simulink model "UnoANFIS"  (R2017a)
settings: Solver=VariableStepAuto  StartTime=0.0  StopTime=1299  RelTol=1e-3
undefined symbols (not defined in the file or in its folder): anfis, anfis3, datos2
libraries: dspsrcs4 x4, fuzblock x1
settings Model: Creator=Dell  LastModifiedBy=Dell

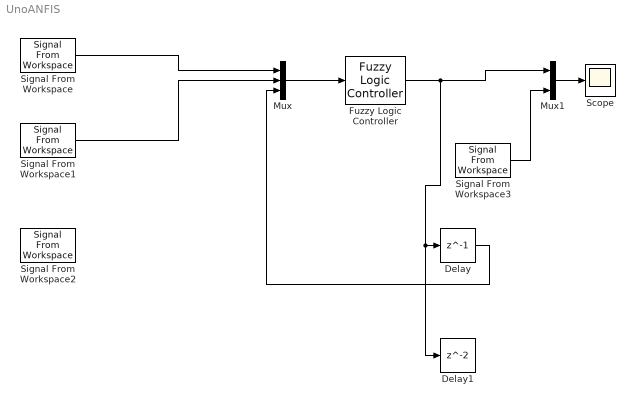
== system UnoANFIS ==
  Delay : Delay  DelayLength=1  InitialCondition=0
  Delay1 : Delay  InitialCondition=0
  Fuzzy Logic Controller : fuzblock/Fuzzy Logic  Controller  fis=[anfis3]
  Mux : Mux  Inputs=3
  Mux1 : Mux  Inputs=2
  Scope : Scope
  Signal From Workspace : dspsrcs4/Signal From Workspace  X=datos2(:,1)  Ts=1  nsamps=1  OutputAfterFinalValue=Setting to zero  ignoreOrWarnInputAndFrameLengths=off  OutputFrames=off
  Signal From Workspace1 : dspsrcs4/Signal From Workspace  X=datos2(:,2)  Ts=1  nsamps=1  OutputAfterFinalValue=Setting to zero  ignoreOrWarnInputAndFrameLengths=off  OutputFrames=off
  Signal From Workspace2 : dspsrcs4/Signal From Workspace  X=anfis(:,3)  Ts=1  nsamps=1  OutputAfterFinalValue=Setting to zero  ignoreOrWarnInputAndFrameLengths=off  OutputFrames=off
  Signal From Workspace3 : dspsrcs4/Signal From Workspace  X=datos2(:,4)  Ts=1  nsamps=1  OutputAfterFinalValue=Setting to zero  ignoreOrWarnInputAndFrameLengths=off  OutputFrames=off
  wires:
  Mux/1 -> Fuzzy Logic Controller/1
  Signal From Workspace/1 -> Mux/1
  Fuzzy Logic Controller/1 -> Delay1/1, Delay/1, Mux1/1
  Signal From Workspace3/1 -> Mux1/2
  Mux1/1 -> Scope/1
  Signal From Workspace1/1 -> Mux/2
  Delay/1 -> Mux/3
